simulink library "ams_primitives"  (R2014b)
settings: Solver=ode45  StartTime=0.0  StopTime=10.0  RelTol=1e-3
undefined symbols (not defined in the file or in its folder): UI
libraries: simulink x5, DesignElements x1, dspbuff3 x1, serdes_modeling x1
settings Model: Creator=Jase  LastModifiedBy=Jase

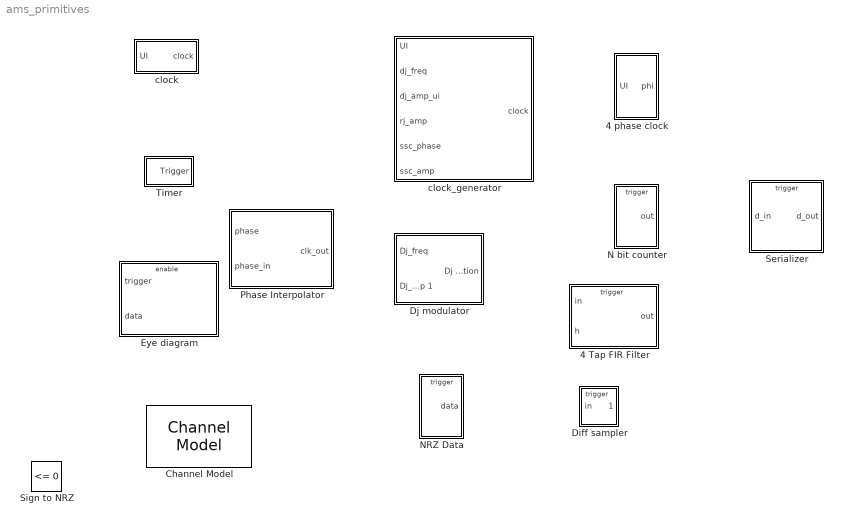
== system ams_primitives ==
  4 Tap FIR Filter : Subsystem
  4 phase clock : Subsystem
  Channel Model : DesignElements/Channel Model  bit_rate=1e9
  Diff sampler : Subsystem
  "Dj modulator " : Subsystem
  Eye diagram : Subsystem  mask{UI=UI, N=100, Num_traces=1000}
      mask prompts: UI "Unit Interval"; N "Number of samples/UI"; Num_traces "Number of traces to record"
  N bit counter : Subsystem  mask{N=4}
      mask prompts: N "Number of bits"
  NRZ Data : Subsystem
  Phase Interpolator : Subsystem  mask{N=128}
      mask prompts: N "Number of PI phases"
  Serializer : Subsystem  mask{N=4}
      mask prompts: N "Simulink:blkprm_prompts:ConstConstValue"
      mask TypeOptions N: Number of bits/Value
  Sign to NRZ : simulink/Logic and Bit Operations/Compare To Zero  relop=<=  OutDataTypeStr=boolean  mask(Compare To Zero){}
  Timer : Subsystem  mask{Time=1e-9}
      mask prompts: Time "Timer value"
  "clock " : Subsystem
  "clock_generator " : Subsystem  Description=A clock generator for performing jitter tolerance simulatons.

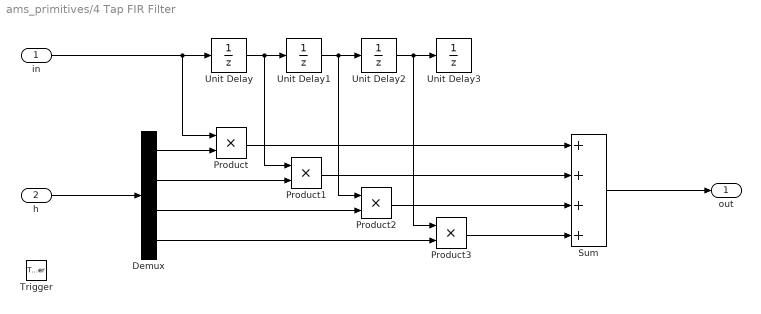
== system ams_primitives/4 Tap FIR Filter ==
  in : Inport
  h : Inport  Port=2
  Trigger : TriggerPort  PortDimensions=1
  Demux : Demux
  Product{,1..3} (4 alike) : Product
  Sum : Sum  Inputs=++++
  Unit Delay{,1..3} (4 alike) : UnitDelay  SampleTime=-1
  out : Outport
  wires:
  Product1/1 -> Sum/2
  Unit Delay/1 -> Unit Delay1/1, Product1/1
  Demux/4 -> Product3/2
  Unit Delay1/1 -> Unit Delay2/1, Product2/1
  h/1 -> Demux/1
  Demux/2 -> Product1/2
  Demux/3 -> Product2/2
  Demux/1 -> Product/2
  Unit Delay2/1 -> Unit Delay3/1, Product3/1
  in/1 -> Unit Delay/1, Product/1
  Sum/1 -> out/1
  Product2/1 -> Sum/3
  Product/1 -> Sum/1
  Product3/1 -> Sum/4

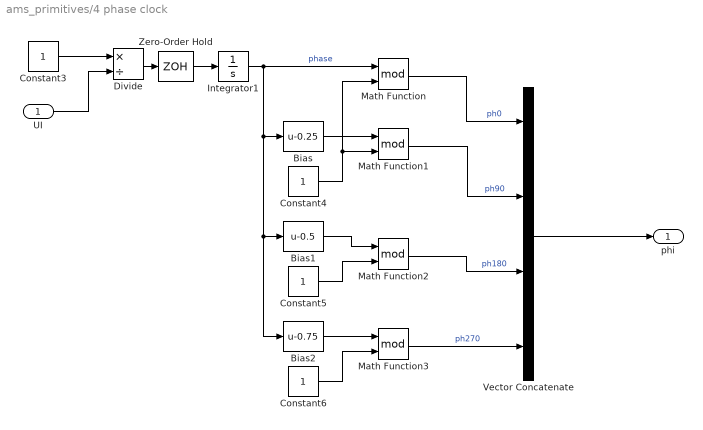
== system ams_primitives/4 phase clock ==
  "UI " : Inport
  Bias : Bias  Bias=-0.25
  Bias1 : Bias  Bias=-0.5
  Bias2 : Bias  Bias=-0.75
  Constant{3..6} (4 alike) : Constant
  Divide : Product  Inputs=*/
  Integrator1 : Integrator
  Math Function{,1..3} (4 alike) : Math  Operator=mod  SaturateOnIntegerOverflow=on
  Vector Concatenate : Concatenate  NumInputs=4
  Zero-Order Hold : ZeroOrderHold  SampleTime=1e-12
  phi : Outport
  wires:
  Vector Concatenate/1 -> phi/1
  Math Function1/1 -> Vector Concatenate/2  "ph90"
  Math Function2/1 -> Vector Concatenate/3  "ph180"
  Math Function3/1 -> Vector Concatenate/4  "ph270"
  Math Function/1 -> Vector Concatenate/1  "ph0"
  Zero-Order Hold/1 -> Integrator1/1
  Bias2/1 -> Math Function3/1
  Integrator1/1 -> Math Function/1, Bias/1, Bias1/1, Bias2/1  "phase"
  Bias1/1 -> Math Function2/1
  Constant5/1 -> Math Function2/2
  Constant6/1 -> Math Function3/2
  Bias/1 -> Math Function1/1
  Constant3/1 -> Divide/1
  Constant4/1 -> Math Function1/2, Math Function/2
  Divide/1 -> Zero-Order Hold/1
  "UI "/1 -> Divide/2

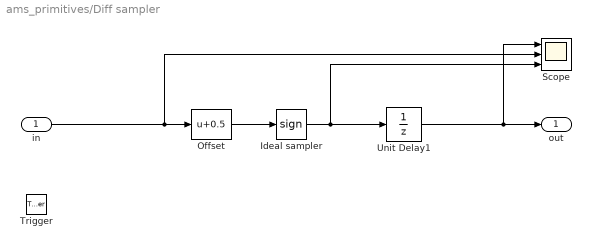
== system ams_primitives/Diff sampler ==
  in : Inport
  Trigger : TriggerPort  PortDimensions=1
  Ideal sampler : Signum
  Offset : Bias  Bias=0.5
  Scope : Scope  NumInputPorts=3
      settings: YMin=-5~-5~-5  YMax=5~5~5  SaveName=ScopeData5
  Unit Delay1 : UnitDelay  SampleTime=-1
  out : Outport
  wires:
  Unit Delay1/1 -> out/1, Scope/1
  in/1 -> Offset/1, Scope/2
  Offset/1 -> Ideal sampler/1
  Ideal sampler/1 -> Unit Delay1/1, Scope/3

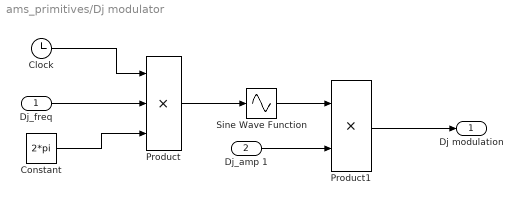
== system ams_primitives/Dj modulator  ==
  "Dj_freq " : Inport
  Dj_amp 1 : Inport  Port=2
  Clock : Clock
  Constant : Constant  Value=2*pi
  Product : Product  Inputs=3
  Product1 : Product
  Sine Wave Function : Sin  TimeSource=Use external signal  SampleTime=0
  Dj modulation : Outport
  wires:
  Product1/1 -> Dj modulation/1
  Product/1 -> Sine Wave Function/1
  Constant/1 -> Product/3
  "Dj_freq "/1 -> Product/2
  Clock/1 -> Product/1
  Dj_amp 1/1 -> Product1/2
  Sine Wave Function/1 -> Product1/1

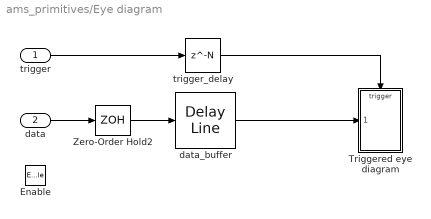
== system ams_primitives/Eye diagram ==
  trigger : Inport
  data : Inport  Port=2
  Enable : EnablePort
  Triggered eye diagram : Subsystem
  Zero-Order Hold2 : ZeroOrderHold  SampleTime=UI/N
  data_buffer : dspbuff3/Delay Line  siz=2*N  ic=0  directfeed=on  enable_output=off  hold_output=off  TreatMby1Signals=One channel
  trigger_delay : Delay  DelayLength=N  SampleTime=UI/N
  wires:
  data/1 -> Zero-Order Hold2/1
  data_buffer/1 -> Triggered eye diagram/1(data_in)
  trigger/1 -> trigger_delay/1
  trigger_delay/1 -> Triggered eye diagram/Trigger
  Zero-Order Hold2/1 -> data_buffer/1

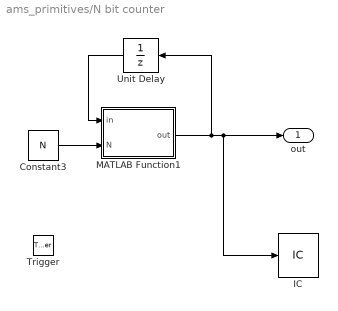
== system ams_primitives/N bit counter ==
  Trigger : TriggerPort  PortDimensions=1
  Constant3 : Constant  Value=N
  IC : InitialCondition  Value=0
  MATLAB Function1 : MATLAB Function  TreatAsAtomicUnit=on
  Unit Delay : UnitDelay  SampleTime=-1
  out : Outport
  wires:
  Unit Delay/1 -> MATLAB Function1/1(in)
  MATLAB Function1/1(out) -> out/1, IC/1, Unit Delay/1
  Constant3/1 -> MATLAB Function1/2(N)

== system ams_primitives/NRZ Data ==
  Trigger : TriggerPort
  Compare To Zero : simulink/Logic and Bit Operations/Compare To Zero  relop=<=  OutDataTypeStr=boolean
  Random Number : RandomNumber
  data : Outport
  wires:
  Random Number/1 -> Compare To Zero/1
  Compare To Zero/1 -> data/1

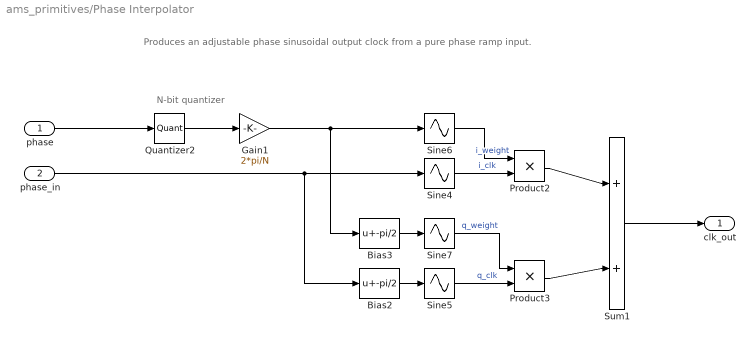
== system ams_primitives/Phase Interpolator ==
  note: Produces an adjustable phase sinusoidal output clock from a pure phase ramp input.
  note: N-bit quantizer
  phase : Inport
  phase_in : Inport  Port=2
  Bias2 : Bias  Bias=-pi/2
  Bias3 : Bias  Bias=-pi/2
  Gain1 : Gain  Gain=2*pi/N
  Product2 : Product
  Product3 : Product
  Quantizer2 : Quantizer  QuantizationInterval=1
  Sine{4..7} (4 alike) : Sin  TimeSource=Use external signal  SampleTime=0
  Sum1 : Sum  Inputs=+|+
  clk_out : Outport
  wires:
  Sine4/1 -> Product2/2  "i_clk"
  Sine5/1 -> Product3/2  "q_clk"
  Product2/1 -> Sum1/1
  Sine7/1 -> Product3/1  "q_weight"
  phase_in/1 -> Sine4/1, Bias2/1
  Bias2/1 -> Sine5/1
  Product3/1 -> Sum1/2
  Gain1/1 -> Sine6/1, Bias3/1
  Sine6/1 -> Product2/1  "i_weight"
  Bias3/1 -> Sine7/1
  phase/1 -> Quantizer2/1
  Quantizer2/1 -> Gain1/1
  Sum1/1 -> clk_out/1

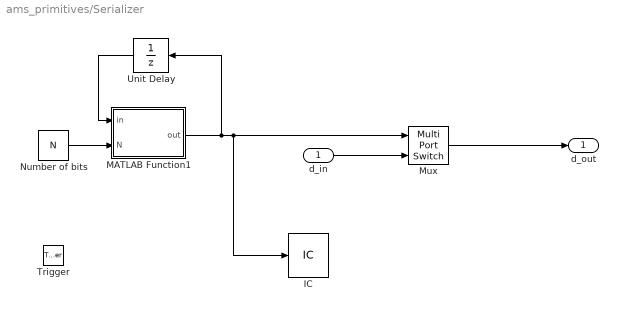
== system ams_primitives/Serializer ==
  d_in : Inport
  Trigger : TriggerPort  PortDimensions=1
  IC : InitialCondition  Value=0
  MATLAB Function1 : MATLAB Function  TreatAsAtomicUnit=on
  Mux : MultiPortSwitch  DataPortOrder=Zero-based contiguous  Inputs=1  zeroidx=on
  Number of bits : Constant  Value=N
  Unit Delay : UnitDelay  SampleTime=-1
  d_out : Outport
  wires:
  Unit Delay/1 -> MATLAB Function1/1(in)
  Number of bits/1 -> MATLAB Function1/2(N)
  MATLAB Function1/1(out) -> IC/1, Mux/1, Unit Delay/1
  d_in/1 -> Mux/2
  Mux/1 -> d_out/1

== system ams_primitives/Timer ==
  Clock : Clock
  Compare To Constant : simulink/Logic and Bit Operations/Compare To Constant  relop=>=  const=Time  OutDataTypeStr=boolean
  Trigger : Outport
  wires:
  Clock/1 -> Compare To Constant/1
  Compare To Constant/1 -> Trigger/1

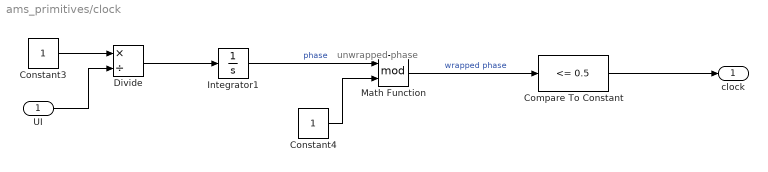
== system ams_primitives/clock  ==
  note: unwrapped phase
  UI : Inport
  Compare To Constant : simulink/Logic and Bit Operations/Compare To Constant  relop=<=  const=0.5  OutDataTypeStr=boolean
  Constant3 : Constant
  Constant4 : Constant
  Divide : Product  Inputs=*/
  Integrator1 : Integrator
  Math Function : Math  Operator=mod  SaturateOnIntegerOverflow=on
  clock : Outport
  wires:
  Compare To Constant/1 -> clock/1
  Math Function/1 -> Compare To Constant/1  "wrapped phase"
  Integrator1/1 -> Math Function/1  "phase"
  Divide/1 -> Integrator1/1
  Constant4/1 -> Math Function/2
  UI/1 -> Divide/2
  Constant3/1 -> Divide/1

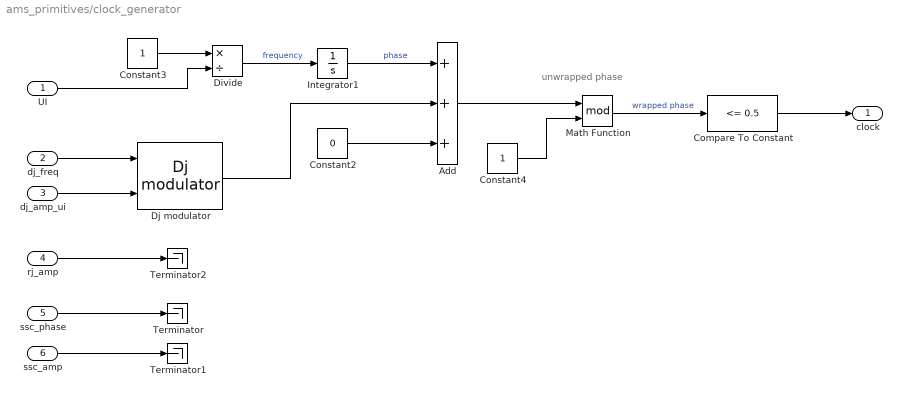
== system ams_primitives/clock_generator  ==
  note: unwrapped phase
  UI : Inport
  dj_freq : Inport  Port=2
  dj_amp_ui : Inport  Port=3
  rj_amp : Inport  Port=4
  ssc_phase : Inport  Port=5
  ssc_amp : Inport  Port=6
  Add : Sum  Inputs=+++
  Compare To Constant : simulink/Logic and Bit Operations/Compare To Constant  relop=<=  const=0.5  OutDataTypeStr=boolean
  Constant2 : Constant  Value=0
  Constant3 : Constant
  Constant4 : Constant
  Divide : Product  Inputs=*/
  "Dj modulator " : serdes_modeling/Dj modulator 
  Integrator1 : Integrator
  Math Function : Math  Operator=mod  SaturateOnIntegerOverflow=on
  Terminator : Terminator
  Terminator1 : Terminator
  Terminator2 : Terminator
  clock : Outport
  wires:
  Integrator1/1 -> Add/1  "phase"
  Constant3/1 -> Divide/1
  Constant2/1 -> Add/3
  UI/1 -> Divide/2
  Constant4/1 -> Math Function/2
  Compare To Constant/1 -> clock/1
  Math Function/1 -> Compare To Constant/1  "wrapped phase"
  ssc_amp/1 -> Terminator1/1
  dj_amp_ui/1 -> "Dj modulator "/2
  Add/1 -> Math Function/1
  Divide/1 -> Integrator1/1  "frequency"
  ssc_phase/1 -> Terminator/1
  rj_amp/1 -> Terminator2/1
  dj_freq/1 -> "Dj modulator "/1
  "Dj modulator "/1 -> Add/2

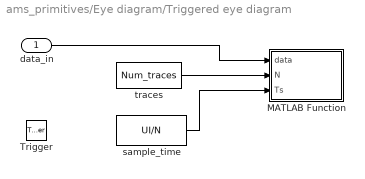
== system ams_primitives/Eye diagram/Triggered eye diagram ==
  data_in : Inport
  Trigger : TriggerPort  PortDimensions=1
  MATLAB Function : MATLAB Function  TreatAsAtomicUnit=on
  sample_time : Constant  Value=UI/N
  traces : Constant  Value=Num_traces
  wires:
  sample_time/1 -> MATLAB Function/3(Ts)
  traces/1 -> MATLAB Function/2(N)
  data_in/1 -> MATLAB Function/1(data)

== matlab function ams_primitives/N bit counter/MATLAB Function1 ==
  data: in input; out output; N input
function out = fcn(in, N)
%#codegen
    if (in == N-1)
        out = 0
    else
        out = in + 1
    end

== matlab function ams_primitives/Serializer/MATLAB Function1 ==
  data: in input; out output; N input
function out = fcn(in, N)
%#codegen
    if (in == N-1)
        out = 0
    else
        out = in + 1
    end

== matlab function ams_primitives/Eye diagram/Triggered eye diagram/MATLAB Function ==
  data: data input; N input; Ts input
function eye_plot( data, N, Ts)
%UNTITLED3 Summary of this function goes here
%   Detailed explanation goes here

    persistent traces;
    persistent line_number;
    persistent first_time;
    persistent x;
    persistent f;
    
    coder.extrinsic('line','set','error','grid');
    
    if (N>1000)
        error('Number of eye traces to plot is limited to 1000');
    end
    
    if isempty(first_time)
        first_time=1;
        f = figure;
        l = length(data)-1;
        x = -l/2:l/2;   
        x = x/Ts;
        traces = ones(1,1000);
        line_number = 0;
    end

    figure(f);
    
    if (first_time == 1)
        xlim([min(x), max(x)]);
        ylabel('Amplitude');
        xlabel('UI');
        grid('on');
        title('Eye diagram');
        alpha(0.02);
        first_time = 0;

        % Fill the plot with transparent lines.  We'll reset
        % their Y data when data comes in from the simulation
        for k=1:N
            h = line('Xdata',x,'Ydata',rand(length(data), 1),'color',[1 0 0 0.0]);
            traces(k)=h;
        end
    end
    index = mod(line_number, N);
    set(traces(index + 1), 'Ydata', data, 'color', [0 0 1 .2]);
    line_number = line_number + 1;  
end
